simulink model "TrayectoriaStateFlow"  (R2023b)
settings: Solver=FixedStepAuto  StartTime=0.0  StopTime=100  RelTol=1e-3  EnableMultiTasking=on
model workspace (MAT data in the model file):
  d = 0.175
settings Model: ExtModeTrigDuration=2  Creator=Enrique  LastModifiedBy=Enrique
settings OptimizationCC: EnhancedBackFolding=on  PassReuseOutputArgsAs=Individual arguments  ZeroExternalMemoryAtStartup=off  ZeroInternalMemoryAtStartup=off  MaxStackSize=64  OptimizeBlockOrder=speed  DifferentSizesBufferReuse=on  EfficientTunableParamExpr=on
settings DebuggingCC: AlgebraicLoopMsg=none  ParameterTunabilityLossMsg=error
settings HardwareCC: ProdBitPerInt=16  ProdBitPerPointer=16  ProdBitPerSizeT=16  ProdBitPerPtrDiffT=16  ProdLargestAtomicFloat=None  ProdWordSize=8  ProdHWDeviceType=Atmel->AVR  UseEmbeddedCoderFeatures=off  UseSimulinkCoderFeatures=off
settings SFSimCC: MATLABDynamicMemAlloc=off
settings RTWCC: Description=Embedded Coder  SystemTargetFile=ert.tlc  HardwareBoard=Arduino Mega 2560  TemplateMakefile=ert_default_tmf  Toolchain=Arduino AVR  BuildConfiguration=Faster Runs
settings CodeAppCC: ForceParamTrailComments=on  IgnoreCustomStorageClasses=off  OperatorAnnotations=on  SimulinkDataObjDesc=on  SFDataObjDesc=on  InsertBlockDesc=on
settings ERTTargetCC: SupportContinuousTime=on  SupportNonInlinedSFcns=on  SupportVariableSizeSignals=on  ExtModeTransport=3  ExtModeStaticAlloc=on  ExtModeAutomaticAllocSize=off  ExtModeStaticAllocSize=2048  ExtModeMexFile=ext_xcp  ExtModeIntrfLevel=Level2 - Open

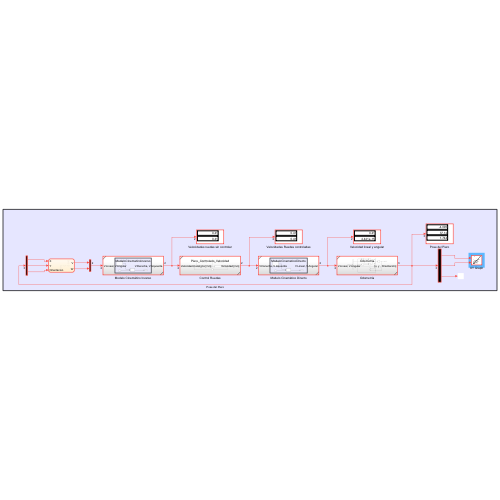
[thumbnail: Simulink's stored preview of the top-level diagram]
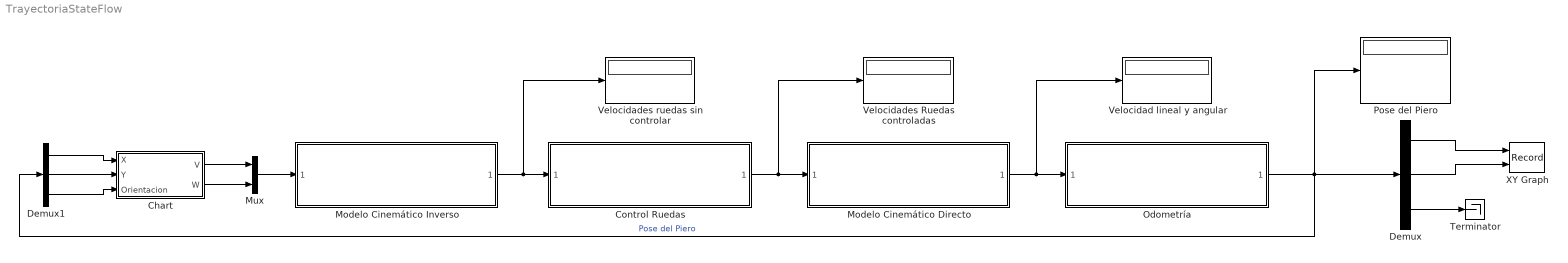
== system TrayectoriaStateFlow ==
  Chart : Stateflow chart  TreatAsAtomicUnit=on
  Control Ruedas : Subsystem  ReferencedSubsystem=Piero_Controlado_Velocidad
  Demux : Demux  Outputs=3
  Demux1 : Demux  Outputs=3
  Modelo Cinemático Directo : Subsystem  ReferencedSubsystem=ModeloCinematicoDirecto
  Modelo Cinemático Inverso : Subsystem  ReferencedSubsystem=ModeloCinematicoInverso
  Mux : Mux  Inputs=2
  Odometría : Subsystem  ReferencedSubsystem=Odometria
  Pose del Piero : Display
  Terminator : Terminator
  Velocidad lineal y angular : Display
  Velocidades Ruedas controladas : Display
  Velocidades ruedas sin controlar : Display
  XY Graph : Record  FileSettingsInternal="{\"entries\":[{\"content\":{\"excelSettings\":{\"content\":{},\"type\":\"Streamout.ExcelSettings\"}},\"type\":\"Streamout.FileSettingStorage\",\"uuid\":\"\"}],\"packageUris\":[\"http:\\/\\/schema.mathworks.com\\/mf0\\/streamout_blocks\\/R2020a\"],\"version\":\"1.0\"}"  Layout=[1 1]  SignalsInternal="{\"entries\":[{\"content\":{\"signals\":[{\"content\":{\"blockPath\":[],\"dimensions\":[1],\"domain\":\"\",\"lineColor\":\"#a2142f\",\"plots\":[ 1 ],\"port\":1,\"sid\":[\"\"],\"signalID\":1,\"signalName\":\"Demux:1\"},\"type\":\"RecordBlkView.Signal\",\"uuid\":\"\"},{\"content\":{\"blockPath\":[],\"dimensions\":[1],\"domain\":\"\",\"lineColor\":\"#139fff\",\"plots\":[ 1 ],\"port\":2,\"sid\":[\"\"],\"signalID\":2,\"signalName\":\"Demux:2\"},\"type\":\"RecordBlkView.Signal\",\"uuid\":\"\"}]},\"type\":\"RecordBlkView.InputSignals\",\"uuid\":\"\"}],\"packageUris\":[\"http:\\/\\/schema.mathworks.com\\/mf0\\/streamout_blocks\\/R2020a\"],\"version\":\"1.0\"}"  VisualizationBindings="{\"xyplotplugin\":{\"info\":[{\"series\":[{\"bindingParametersList\":[{\"parameter\":\"X-Axis\",\"signalID\":1,\"signalName\":\"Demux:1\"},{\"parameter\":\"Y-Axis\",\"signalID\":2,\"signalName\":\"Demux:2\"}],\"seriesID\":0}],\"subplotID\":1}]}}"  CompatibilityTag=XY
  wires:
  Modelo Cinemático Inverso/1 -> Velocidades ruedas sin controlar/1, Control Ruedas/1
  Control Ruedas/1 -> Velocidades Ruedas controladas/1, Modelo Cinemático Directo/1
  Modelo Cinemático Directo/1 -> Velocidad lineal y angular/1, Odometría/1
  Odometría/1 -> Pose del Piero/1, Demux1/1, Demux/1  "Pose del Piero"
  Demux/2 -> XY Graph/2
  Demux/1 -> XY Graph/1
  Demux/3 -> Terminator/1
  Chart/1(V) -> Mux/1
  Chart/2(W) -> Mux/2
  Mux/1 -> Modelo Cinemático Inverso/1
  Demux1/1 -> Chart/1(X)
  Demux1/2 -> Chart/2(Y)
  Demux1/3 -> Chart/3(Orientacion)

== stateflow chart TrayectoriaStateFlow/Chart ==
  state Fin
    V = 0;
    W = 0;
  state AvanceRecto4
    V = 0.41;
    W = 0;
  state GiroDerecha
    V = 0.2;
    W = -pi/4;
  state AvanceRecto3
    V = 0.41;
    W = 0;
  state GiroIzquierda2
    V = 0.2;
    W = pi/4;
  state AvanceRecto2
    V = 0.41;
    W = 0;
  state AvanceRecto
    V = 0.41;
    W = 0;
  state GiroIzquierda
    V = 0.2;
    W = pi/4;
  state Inicio
    V = 0;
    W = 0;
  AvanceRecto4 -> Fin : [Y > 14]
  GiroIzquierda2 -> AvanceRecto4 : [Orientacion > pi/2]
  GiroDerecha -> AvanceRecto3 : [Orientacion > 0]
  AvanceRecto3 -> GiroIzquierda2 : [X > 3]
  AvanceRecto2 -> GiroDerecha : [Y > 12]
  GiroIzquierda -> AvanceRecto2 : [Orientacion > pi/2]
  (default) -> Inicio
  AvanceRecto -> GiroIzquierda : [X > 2.1]
  Inicio -> AvanceRecto : after(1,sec)
  data: V output; W output; X input; Y input; Orientacion input
